simulink model "mpc_miso"  (Simulink 6.0)
settings: Solver=ode45  SolverMode=SingleTasking  StartTime=0.0  StopTime=Tstop  RelTol=1e-3
values from neighbouring files (symbols this model uses):
  A = sys.a    [misosim.m]    (also in mpcutarget.m)
  B = sys.b    [misosim.m]    (also in mpcutarget.m)
  C = sys.c    [misosim.m]    (also in mpcutarget.m)
  D = sys.d    [misosim.m]    (also in mpcutarget.m)
libraries: mpclib x1
settings Model: Creator=jowen  LastModifiedBy=jowen  ExtModeTrigMode=oneshot  ExtModeArmWhenConnect=off
settings DataIOCC: LimitDataPoints=off  SignalLoggingName=sigsOut
settings OptimizationCC: BooleanDataType=off
settings DebuggingCC: CheckExecutionContextPreStartOutputMsg=on  CheckExecutionContextRuntimeOutputMsg=on  SolverPrmCheckMsg=none  IntegerOverflowMsg=none
settings HardwareCC: TargetUnknown=on
settings SFSimCC: SFSimApplyToAllLibs=on  SFSimBuildMode=Incremental

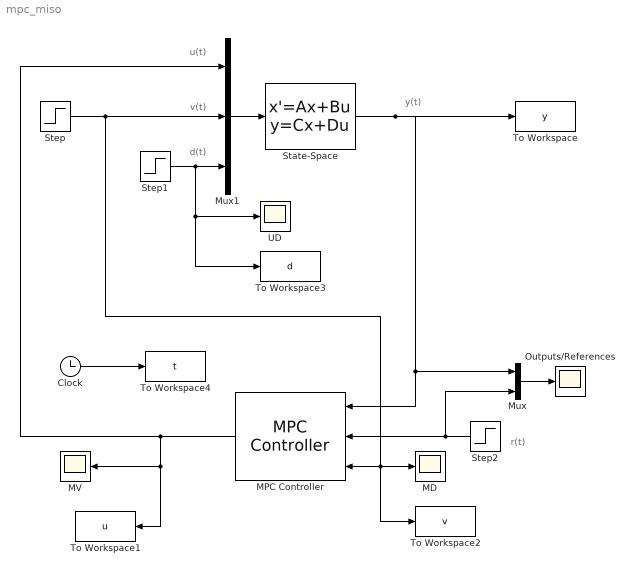
== system mpc_miso ==
  note: u(t)
  note: y(t)
  note: r(t)
  note: v(t)
  note: d(t)
  Clock : Clock
      settings: Decimation=10
  MD : Scope
      settings: TimeRange=30  YMin=0  YMax=1  DataFormat=Structure
  MPC Controller : mpclib/MPC Controller  Orientation=left  mpcobj=MPCobj  n_mv=0  x0=[]  ref_from_ws=off  ref_signal_name=[]  ref_preview=on  md_from_ws=off  md_signal_name=[]  md_preview=on  from_project=off  md_inport=on  project_file=MPCtask.mat
  MV : Scope
      settings: TimeRange=30  YMin=-0.5  YMax=1.5  DataFormat=Structure
  Mux : Mux  Inputs=2
  Mux1 : Mux  Inputs=3
  Outputs/References : Scope
      settings: TimeRange=30  YMin=0  YMax=1.5  DataFormat=Structure
  State-Space : StateSpace  A=A  B=B  C=C  D=D  X0=[0 0 0 0 0]'
  Step : Step  Time=10  SampleTime=0
  Step1 : Step  Time=20  After=-.5  SampleTime=0
  Step2 : Step  Orientation=left  Time=0  SampleTime=0
  To Workspace : ToWorkspace  VariableName=y  SampleTime=-1  SaveFormat=Array
      settings: MaxDataPoints=Inf
  To Workspace1 : ToWorkspace  VariableName=u  SampleTime=-1  SaveFormat=Array
      settings: MaxDataPoints=Inf
  To Workspace2 : ToWorkspace  VariableName=v  SampleTime=-1  SaveFormat=Array
      settings: MaxDataPoints=Inf
  To Workspace3 : ToWorkspace  VariableName=d  SampleTime=-1  SaveFormat=Array
      settings: MaxDataPoints=Inf
  To Workspace4 : ToWorkspace  VariableName=t  SampleTime=-1  SaveFormat=Array
      settings: MaxDataPoints=Inf
  UD : Scope
      settings: TimeRange=30  YMin=-0.5  YMax=0  DataFormat=Structure
  wires:
  Mux1/1 -> State-Space/1
  Mux/1 -> Outputs/References/1
  Step2/1 -> Mux/2, MPC Controller/2
  State-Space/1 -> To Workspace/1, Mux/1, MPC Controller/1
  Step1/1 -> Mux1/3, UD/1, To Workspace3/1
  Step/1 -> Mux1/2, To Workspace2/1, MD/1, MPC Controller/3
  MPC Controller/1 -> Mux1/1, MV/1, To Workspace1/1
  Clock/1 -> To Workspace4/1
